simulink model "transmission_system_healthy"  (R2025b)
settings: Solver=FixedStepAuto  StartTime=0.0  StopTime=5/60  FixedStep=1/3840  RelTol=1e-3
settings Model: Creator=faizshaikh  LastModifiedBy=faizshaikh

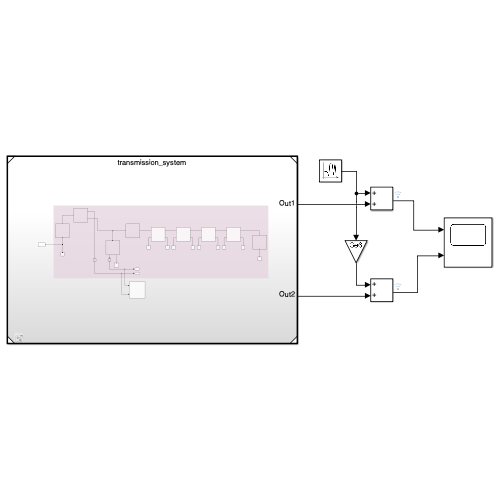
[thumbnail: Simulink's stored preview of the top-level diagram]
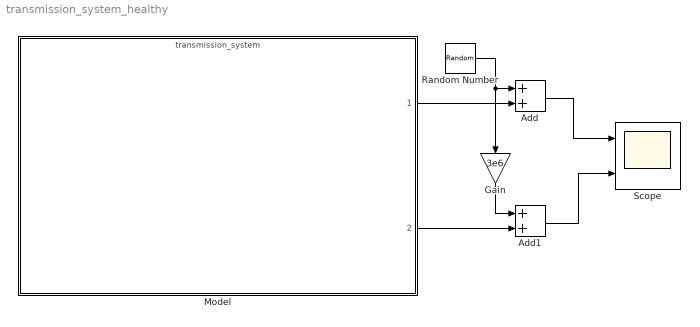
== system transmission_system_healthy ==
  Add : Sum
  Add1 : Sum
  Gain : Gain  Gain=3e6
  Model : ModelReference  ModelNameDialog=transmission_system.slx  SimulationMode=Normal  ModelReferenceVersion=1.15
  Random Number : RandomNumber  Variance=1e-9  SampleTime=1/3840
  Scope : Scope  NumInputPorts=2
      settings: ActiveDisplayYMinimum=-0.00297499770433086  ActiveDisplayYMaximum=0.0025251412579341791
  wires:
  Model/1 -> Add/2
  Random Number/1 -> Gain/1, Add/1
  Add/1 -> Scope/1
  Model/2 -> Add1/2
  Add1/1 -> Scope/2
  Gain/1 -> Add1/1
